simulink model "ex6sima"  (R2015a)
settings: Solver=ode3  StartTime=0.0  StopTime=100  FixedStep=0.01  RelTol=1e-3
values from neighbouring files (symbols this model uses):
  Cden = Cden'    [ex6.m]    (also in runsim.m)
  Cnum = Cnum'    [ex6.m]    (also in runsim.m)
  den = Gs.den{1}    [ex6.m]    (also in s2z.m = G.den{1}')
  num = Gs.num{1}    [ex6.m]    (also in s2z.m = G.num{1}')
  Ts = Ts1    (= 0.25)    [ex6.m]
settings Model: Creator=brunopeixoto  LastModifiedBy=brunopeixoto

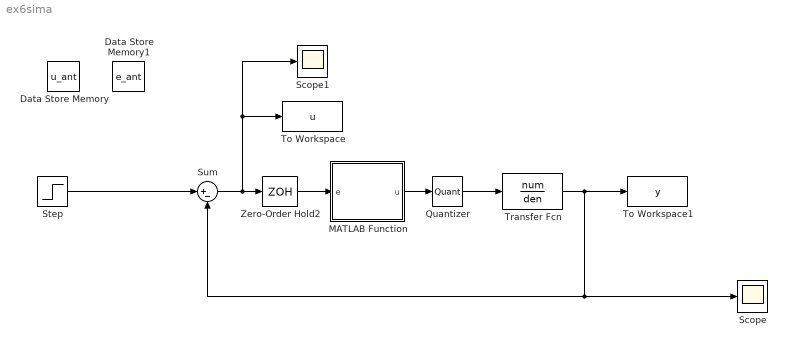
== system ex6sima ==
  Data Store Memory : DataStoreMemory  DataStoreName=u_ant  InitialValue=u0  OutDataTypeStr=double
  Data Store Memory1 : DataStoreMemory  DataStoreName=e_ant  InitialValue=e0  OutDataTypeStr=double
  MATLAB Function : MATLAB Function  TreatAsAtomicUnit=on  SystemSampleTime=Ts
  Quantizer : Quantizer  QuantizationInterval=0.01
  Scope : Scope
  Scope1 : Scope
  Step : Step  Time=0  SampleTime=Ts
  Sum : Sum  Inputs=|+-
  To Workspace : ToWorkspace  VariableName=u  SampleTime=-1
      settings: Save2DSignal=2-D array (concatenate along first dimension)
  To Workspace1 : ToWorkspace  VariableName=y  SampleTime=-1
      settings: Save2DSignal=2-D array (concatenate along first dimension)
  Transfer Fcn : TransferFcn  Numerator=num  Denominator=den
  Zero-Order Hold2 : ZeroOrderHold  SampleTime=Ts
  wires:
  MATLAB Function/1(u) -> Quantizer/1
  Quantizer/1 -> Transfer Fcn/1
  Transfer Fcn/1 -> Scope/1, Sum/2, To Workspace1/1
  Step/1 -> Sum/1
  Sum/1 -> Scope1/1, To Workspace/1, Zero-Order Hold2/1
  Zero-Order Hold2/1 -> MATLAB Function/1(e)

== matlab function ex6sima/MATLAB Function ==
  settings: updateMethod=DISCRETE  sampleTime=Ts
  data: e input; u output size=1; Cnum parameter; u_ant data_store_memory; Cden parameter; e_ant data_store_memory
function u = fcn(e, Cnum, Cden)
    global u_ant; 
    global e_ant;
    
    if isempty(u_ant)
        q = length(Cden);
        u_ant = zeros(q-1, 1);
    end

    if isempty(e_ant)
        q = length(Cnum);
        e_ant = zeros(q, 1);
    end
    
    m = length(Cnum);
    n = length(Cden);
    
    a = Cnum;
    b = Cden;

    e_ant(1:end-1) = e_ant(2:end);
    e_ant(end) = e;
    
    u = (b'*e_ant - a(2:end)'*u_ant)/a(1);
        
    u_ant(1:end-1) = u_ant(2:end);
    u_ant(end) = u;
end
